simulink model "rotor_dysim"  (R2023b)
settings: Solver=VariableStepAuto  StartTime=0.0  StopTime=10.0  RelTol=1e-3
values from neighbouring files (symbols this model uses):
  C_d0 = 0.01    [rotor_dy.m]
  C_Lalpha = 5.7    [rotor_dy.m]
  omega = Omega    (= 300)    [rotor_dy.m]
  R = 0.5    [rotor_dy.m]
  rho = 1.225    [rotor_dy.m]
  sigma = 0.1    [rotor_dy.m]
  theta_0 = 0.1    [rotor_dy.m]
settings Model: Creator=arya  LastModifiedBy=arya

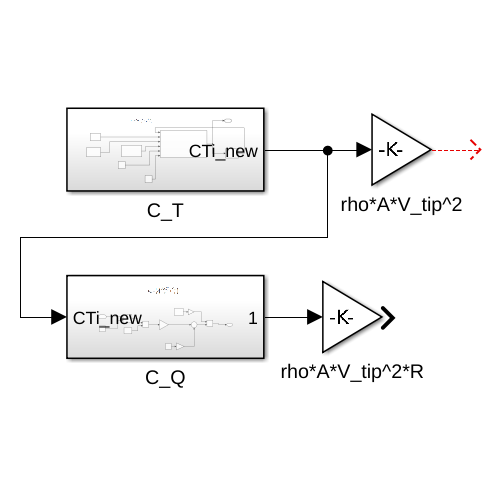
[thumbnail: Simulink's stored preview of the top-level diagram]
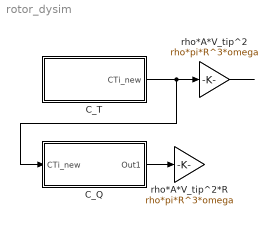
== system rotor_dysim ==
  C_Q : Subsystem
  C_T : Subsystem
  rho*A*V_tip^2 : Gain  Gain=rho*pi*R^3*omega
  rho*A*V_tip^2*R : Gain  Gain=rho*pi*R^3*omega
  wires:
  C_T/1(CTi_new) -> rho*A*V_tip^2/1, C_Q/1(CTi_new)
  rho*A*V_tip^2/1 -> ?
  C_Q/1(Out1) -> rho*A*V_tip^2*R/1

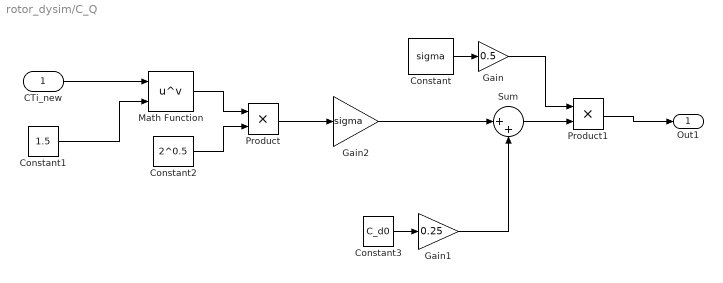
== system rotor_dysim/C_Q ==
  CTi_new : Inport
  Constant : Constant  Value=sigma
  Constant1 : Constant  Value=1.5
  Constant2 : Constant  Value=2^0.5
  Constant3 : Constant  Value=C_d0
  Gain : Gain  Gain=0.5
  Gain1 : Gain  Gain=0.25
  Gain2 : Gain  Gain=sigma
  Math Function : Math  Operator=pow
  Product : Product
  Product1 : Product
  Sum : Sum  Inputs=|++
  Out1 : Outport
  wires:
  Constant/1 -> Gain/1
  CTi_new/1 -> Math Function/1
  Constant1/1 -> Math Function/2
  Math Function/1 -> Product/1
  Constant2/1 -> Product/2
  Product/1 -> Gain2/1
  Constant3/1 -> Gain1/1
  Gain1/1 -> Sum/2
  Gain2/1 -> Sum/1
  Gain/1 -> Product1/1
  Sum/1 -> Product1/2
  Product1/1 -> Out1/1

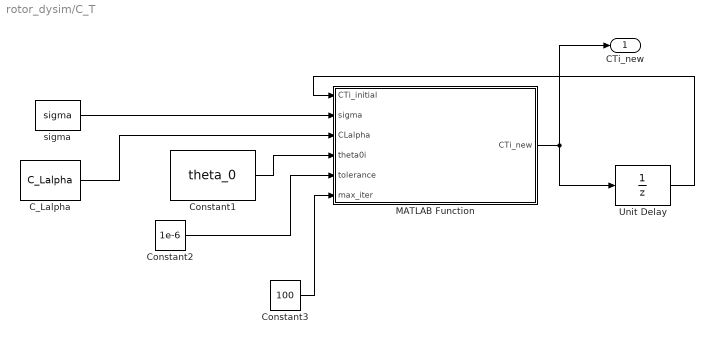
== system rotor_dysim/C_T ==
  C_Lalpha : Constant  Value=C_Lalpha
  Constant1 : Constant  Value=theta_0
  Constant2 : Constant  Value=1e-6
  Constant3 : Constant  Value=100
  MATLAB Function : MATLAB Function  TreatAsAtomicUnit=on
  Unit Delay : UnitDelay  InitialCondition=.05  SampleTime=-1  HasFrameUpgradeWarning=on
  sigma : Constant  Value=sigma
  CTi_new : Outport
  wires:
  C_Lalpha/1 -> MATLAB Function/3(CLalpha)
  sigma/1 -> MATLAB Function/2(sigma)
  Constant1/1 -> MATLAB Function/4(theta0i)
  Constant3/1 -> MATLAB Function/6(max_iter)
  Constant2/1 -> MATLAB Function/5(tolerance)
  MATLAB Function/1(CTi_new) -> Unit Delay/1, CTi_new/1
  Unit Delay/1 -> MATLAB Function/1(CTi_initial)

== matlab function rotor_dysim/C_T/MATLAB Function ==
  data: CTi_initial input; CTi_new output; sigma input; CLalpha input; theta0i input; tolerance input; max_iter input
function CTi_new = newton_raphson_CTi(CTi_initial, sigma, CLalpha, theta0i, tolerance, max_iter)
    % Newton-Raphson method to solve for CTi iteratively

    % Initial guess for CTi
    CTi_old = CTi_initial;

    % Start the iteration process
    for iter = 1:max_iter
        % Calculate the function value
        f_CTi = CTi_old - 0.5 * sigma * CLalpha * (theta0i/3 - 0.5 * sqrt(CTi_old / 2));

        % Calculate the derivative of the function
        df_CTi = 1 + (0.125 * sigma * CLalpha) / sqrt(2*CTi_old);

        % Update the guess using Newton-Raphson formula
        CTi_new = CTi_old - f_CTi / df_CTi;

        % Check for convergence
        if abs(CTi_new - CTi_old) < tolerance
            break;
        end

        % Update CTi_old for the next iteration
        CTi_old = CTi_new;
    end

    % If the maximum number of iterations was reached without convergence
    if iter == max_iter
        warning('Newton-Raphson did not converge within the maximum number of iterations');
    end
end
